simulink model "cartpole"  (R2022a)
settings: Solver=VariableStepAuto  StartTime=0.0  StopTime=10.0  RelTol=1e-3
settings Model: Creator=jack  LastModifiedBy=jack

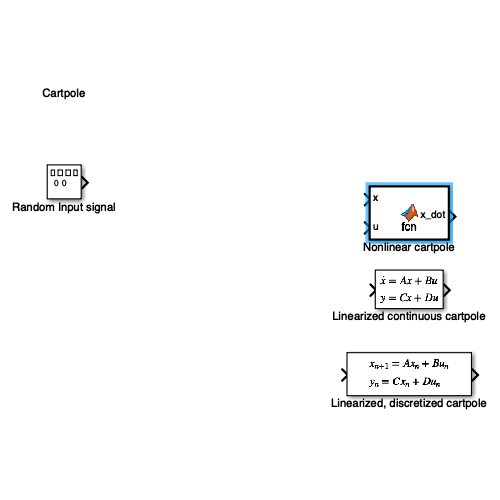
[thumbnail: Simulink's stored preview of the top-level diagram]
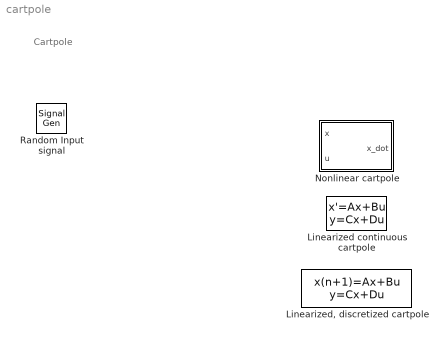
== system cartpole ==
  note: Cartpole
  Linearized continuous cartpole : StateSpace  InitialCondition=0
  "Linearized, discretized cartpole" : DiscreteStateSpace  SampleTime=-1
  Nonlinear cartpole : MATLAB Function  TreatAsAtomicUnit=on
  Random Input signal : SignalGenerator  WaveForm=random  Amplitude=10  Units=rad/sec

== matlab function cartpole/Nonlinear cartpole ==
  data: x input; u input; x_dot output
function x_dot = fcn(x, u)    
    % parameters
    g=9.81;
    m_c= 1.0;
    m_p = 0.1;
    length = 0.5;
    mu_c= 0.0;
    mu_p = 0.01;
    % states
    x2 = x(2);x3 = x(3);x4 = x(4);

    % nonlinear differential equation
    x_dot = zeros(4,1);
    x_dot(4) = ( ...
        g * sin(x3) ...
        + cos(x3) ...
        * ( ...
            ( ...
                -u ...
                - m_p * length * x4^2 * sin(x3) ...
                + mu_c * sign(x2) ...
            ) ...
            / (m_c + m_p) ...
        ) ...
        - (mu_p * x4) / (m_p * length) ...
    ) / ( ...
        length ...
        * (4 / 3 - (m_p * cos(x3)^2) / (m_c + m_p)) ...
    );
    x_dot(1) = x2;
    x_dot(2) = ( ...
        u ...
        + m_p * length * x4^2 * sin(x3) ...
        - m_p * length * x_dot(4) * cos(x3) ...
        - mu_c * sign(x2) ...
    ) / (m_c + m_p);
    x_dot(3) = x4;
